simulink model "S_fuell"  (Simulink 2.00)
settings: Solver=ode45  StartTime=0.0  StopTime=50  MaxStep=0.010  RelTol=1e-3  AbsTol=1e-6
values from neighbouring files (symbols this model uses):
  A1 = 2    [torce11.m]    (also in torcell.mat; waag11.mat)
  A12 = 0.1    [torce11.m]    (also in torcell.mat; waag11.mat)
  A2 = 2    [torce11.m]    (also in torcell.mat; waag11.mat)
  g = 9.8    [ident21.mat]    (also in torce11.m = 9.81; torcell.mat = 9.81; waag11.m = 9.81; waag11.mat = 9.81)
settings Model: SaveTime=off  SaveOutput=off  ConsistencyChecking=off

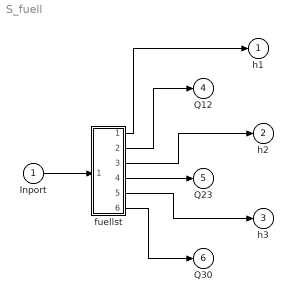
== system S_fuell ==
  Inport : Inport  Port=1  PortWidth=-1  SampleTime=-1
  "fuellst " : Subsystem
  h1 : Outport  Port=1  InitialOutput=0
  h2 : Outport  Port=2  InitialOutput=0
  h3 : Outport  Port=3  InitialOutput=0
  Q12 : Outport  Port=4  InitialOutput=0
  Q23 : Outport  Port=5  InitialOutput=0
  Q30 : Outport  Port=6  InitialOutput=0
  wires:
  Inport/1 -> "fuellst "/1(in_1)
  "fuellst "/6(out_6) -> Q30/1
  "fuellst "/4(out_2) -> Q23/1
  "fuellst "/2(out_3) -> Q12/1
  "fuellst "/5(out_4) -> h3/1
  "fuellst "/3(out_5) -> h2/1
  "fuellst "/1(out_1) -> h1/1

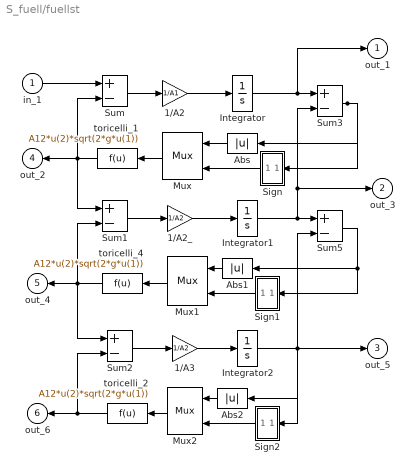
== system S_fuell/fuellst  ==
  in_1 : Inport  Port=1  PortWidth=-1  SampleTime=-1
  1/A2 : Gain  Gain=1/A1
  1/A2_ : Gain  Gain=1/A2
  1/A3 : Gain  Gain=1/A2
  Abs : Abs  Orientation=left
  Abs1 : Abs  Orientation=left
  Abs2 : Abs  Orientation=left
  Integrator : Integrator  ExternalReset=none  InitialConditionSource=internal  InitialCondition=0  LimitOutput=off  UpperSaturationLimit=inf  LowerSaturationLimit=-inf  ShowSaturationPort=off  ShowStatePort=off  AbsoluteTolerance=auto
  Integrator1 : Integrator  ExternalReset=none  InitialConditionSource=internal  InitialCondition=0  LimitOutput=off  UpperSaturationLimit=inf  LowerSaturationLimit=-inf  ShowSaturationPort=off  ShowStatePort=off  AbsoluteTolerance=auto
  Integrator2 : Integrator  ExternalReset=none  InitialConditionSource=internal  InitialCondition=0  LimitOutput=off  UpperSaturationLimit=inf  LowerSaturationLimit=-inf  ShowSaturationPort=off  ShowStatePort=off  AbsoluteTolerance=auto
  Mux : Mux  Orientation=left  Inputs=2
  Mux1 : Mux  Orientation=left  Inputs=2
  Mux2 : Mux  Orientation=left  Inputs=2
  Sign : Subsystem  Orientation=left
      mask Type: Sign
      mask Description: y = sign(x)
      mask Help: Sign Function:\n\t\t\ty = 1 if x > 0\n\t\t\ty = 0 if x = 0\n\t\t\ty = -1 if x < 0
      mask Display: plot(-50,-50,50,50,[-50,50],[0,0],[0,0],[-50,50],[-40,0],[-30,-30],[0,40],[30,30])
  Sign1 : Subsystem  Orientation=left
      mask Type: Sign
      mask Description: y = sign(x)
      mask Help: Sign Function:\n\t\t\ty = 1 if x > 0\n\t\t\ty = 0 if x = 0\n\t\t\ty = -1 if x < 0
      mask Display: plot(-50,-50,50,50,[-50,50],[0,0],[0,0],[-50,50],[-40,0],[-30,-30],[0,40],[30,30])
  Sign2 : Subsystem  Orientation=left
      mask Type: Sign
      mask Description: y = sign(x)
      mask Help: Sign Function:\n\t\t\ty = 1 if x > 0\n\t\t\ty = 0 if x = 0\n\t\t\ty = -1 if x < 0
      mask Display: plot(-50,-50,50,50,[-50,50],[0,0],[0,0],[-50,50],[-40,0],[-30,-30],[0,40],[30,30])
  Sum{,1..3,5} (5 alike) : Sum  Inputs=+-
  toricelli_1 : Fcn  Orientation=left  Expr=A12*u(2)*sqrt(2*g*u(1))
  toricelli_2 : Fcn  Orientation=left  Expr=A12*u(2)*sqrt(2*g*u(1))
  toricelli_4 : Fcn  Orientation=left  Expr=A12*u(2)*sqrt(2*g*u(1))
  out_1 : Outport  Port=1  InitialOutput=0
  out_3 : Outport  Port=2  InitialOutput=0
  out_5 : Outport  Port=3  InitialOutput=0
  out_2 : Outport  Orientation=left  Port=4  InitialOutput=0
  out_4 : Outport  Orientation=left  Port=5  InitialOutput=0
  out_6 : Outport  Orientation=left  Port=6  InitialOutput=0
  wires:
  Integrator/1 -> out_1/1, Sum3/1
  toricelli_2/1 -> out_6/1, Sum2/2
  in_1/1 -> Sum/1
  Sum/1 -> 1/A2/1
  Sum1/1 -> 1/A2_/1
  Sum2/1 -> 1/A3/1
  1/A2/1 -> Integrator/1
  1/A2_/1 -> Integrator1/1
  1/A3/1 -> Integrator2/1
  Integrator1/1 -> out_3/1, Sum3/2, Sum5/1
  toricelli_1/1 -> out_2/1, Sum/2, Sum1/1
  Sum3/1 -> Abs/1, Sign/1(in_1)
  Abs/1 -> Mux/1
  Mux/1 -> toricelli_1/1
  Sign/1(out_1) -> Mux/2
  Mux1/1 -> toricelli_4/1
  Sign1/1(out_1) -> Mux1/2
  Sum5/1 -> Sign1/1(in_1), Abs1/1
  Abs1/1 -> Mux1/1
  toricelli_4/1 -> out_4/1, Sum1/2, Sum2/1
  Abs2/1 -> Mux2/1
  Mux2/1 -> toricelli_2/1
  Sign2/1(out_1) -> Mux2/2
  Integrator2/1 -> out_5/1, Sum5/2, Abs2/1, Sign2/1(in_1)

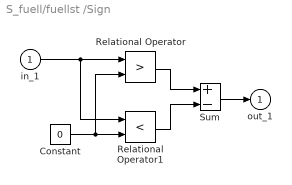
== system S_fuell/fuellst /Sign ==
  in_1 : Inport  Port=1  PortWidth=-1  SampleTime=-1
  Constant : Constant  Value=0
  Relational Operator : RelationalOperator  Operator=>
  Relational Operator1 : RelationalOperator  Operator=<
  Sum : Sum  Inputs=+-
  out_1 : Outport  Port=1  InitialOutput=0
  wires:
  Sum/1 -> out_1/1
  Relational Operator/1 -> Sum/1
  Relational Operator1/1 -> Sum/2
  Constant/1 -> Relational Operator/2, Relational Operator1/2
  in_1/1 -> Relational Operator1/1, Relational Operator/1

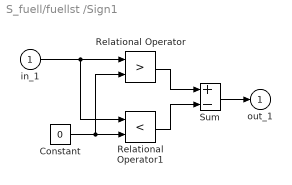
== system S_fuell/fuellst /Sign1 ==
  in_1 : Inport  Port=1  PortWidth=-1  SampleTime=-1
  Constant : Constant  Value=0
  Relational Operator : RelationalOperator  Operator=>
  Relational Operator1 : RelationalOperator  Operator=<
  Sum : Sum  Inputs=+-
  out_1 : Outport  Port=1  InitialOutput=0
  wires:
  Sum/1 -> out_1/1
  Relational Operator/1 -> Sum/1
  Relational Operator1/1 -> Sum/2
  Constant/1 -> Relational Operator/2, Relational Operator1/2
  in_1/1 -> Relational Operator1/1, Relational Operator/1

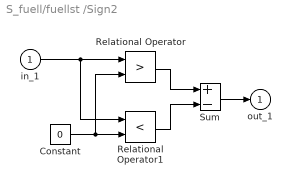
== system S_fuell/fuellst /Sign2 ==
  in_1 : Inport  Port=1  PortWidth=-1  SampleTime=-1
  Constant : Constant  Value=0
  Relational Operator : RelationalOperator  Operator=>
  Relational Operator1 : RelationalOperator  Operator=<
  Sum : Sum  Inputs=+-
  out_1 : Outport  Port=1  InitialOutput=0
  wires:
  Sum/1 -> out_1/1
  Relational Operator/1 -> Sum/1
  Relational Operator1/1 -> Sum/2
  Constant/1 -> Relational Operator/2, Relational Operator1/2
  in_1/1 -> Relational Operator1/1, Relational Operator/1
